simulink library "StatemachineMARCH"  (R2016b)
settings: Solver=VariableStepAuto  StartTime=0.0  StopTime=10.0  RelTol=1e-3
settings Model: Creator=Nathan  LastModifiedBy=march

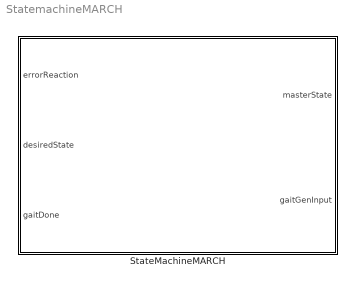
== system StatemachineMARCH ==
  StateMachineMARCH : Stateflow chart  TreatAsAtomicUnit=on

== stateflow chart StatemachineMARCH/StateMachineMARCH ==
  state MASTER_SHUTDOWN
    en: masterState = ExoskeletonState.SHUTTING_DOWN;
  state OPERATION
    state SLOPEUP
      en: masterState = ExoskeletonState.SLOPEUP;
      state startRightSlopeUp
        en: gaitGenInput.targetLeg = Leg.RIGHT;
        %Both leg vectors play at the same time so this only determines
        %what leg starts the stairs step.
        % Leg.Right = Right leg starts stairs step
        % Leg.Left = Left leg starts stair step
        en: gaitGenInput.stepType = StepType.SLOPEUPSTEP;
      state WAIT_SLOPEUP
        en: masterState = ExoskeletonState.SLOPEUP;
        en: gaitGenInput.stepType = StepType.WAITSLOPEUP;
        en: gaitGenInput.targetLeg = Leg.BOTH;
      state INITIALIZE_SLOPEUP
        en: masterState = ExoskeletonState.SLOPEUP;
        en: gaitGenInput.stepType = StepType.INITIALIZESLOPEUP;
        en: gaitGenInput.targetLeg = Leg.BOTH;
      WAIT_SLOPEUP -> startRightSlopeUp [order 1] : [gaitDone]
      INITIALIZE_SLOPEUP -> WAIT_SLOPEUP : [gaitDone]
    state FULLMANUAL
      en: masterState = ExoskeletonState.FULLMANUAL;
    state MANUAL
      en: masterState = ExoskeletonState.MANUAL;
      en: gaitGenInput.targetLeg=Leg.NONE;
      en: gaitGenInput.stepType=StepType.NOSTEP;
    state HOLDSOFA
      en: masterState = ExoskeletonState.HOLDSOFA;
      en: gaitGenInput.stepType = StepType.HOMESOFA;
      en: gaitGenInput.targetLeg = Leg.BOTH;
    state HOLDSIT
      en: masterState = ExoskeletonState.HOLDSIT;
      en: gaitGenInput.stepType = StepType.HOMESIT;
      en: gaitGenInput.targetLeg = Leg.BOTH;
    state STANDUPPROCEDURE
      state INITIALIZE_STANDUP
        en: masterState = ExoskeletonState.STANDINGUP;
        en: gaitGenInput.stepType = StepType.INITIALIZESTANDUP;
        en: gaitGenInput.targetLeg = Leg.BOTH;
      state WAIT_STANDUP
        en: masterState = ExoskeletonState.STANDINGUP;
        en: gaitGenInput.stepType = StepType.WAITSTANDUP;
        en: gaitGenInput.targetLeg = Leg.BOTH;
      state STANDUP
        en: masterState = ExoskeletonState.STANDINGUP;
        en: gaitGenInput.stepType = StepType.STANDUP;
        en: gaitGenInput.targetLeg = Leg.BOTH;
      INITIALIZE_STANDUP -> WAIT_STANDUP : [gaitDone]
      WAIT_STANDUP -> STANDUP [order 2] : [desiredState==ExoskeletonState.HOLDSTAND & gaitDone]
    state SITDOWNPROCEDURE
      state SITDOWN
        en: masterState = ExoskeletonState.SITTINGDOWN;
        en: gaitGenInput.stepType = StepType.SITDOWN;
        en: gaitGenInput.targetLeg = Leg.BOTH;
      state WAIT_SITDOWN
        en: masterState = ExoskeletonState.SITTINGDOWN;
        en: gaitGenInput.stepType = StepType.WAITSITDOWN;
        en: gaitGenInput.targetLeg = Leg.BOTH;
      state INITIALIZE_SITDOWN
        en: masterState = ExoskeletonState.SITTINGDOWN;
        en: gaitGenInput.stepType = StepType.INITIALIZESITDOWN;
        en: gaitGenInput.targetLeg = Leg.BOTH;
      WAIT_SITDOWN -> SITDOWN [order 1] : [desiredState==ExoskeletonState.HOLDSIT & gaitDone]
      INITIALIZE_SITDOWN -> WAIT_SITDOWN : [gaitDone]
    state SOFADOWNPROCEDURE
      state SOFADOWN
        en: masterState = ExoskeletonState.SOFADOWN;
        en: gaitGenInput.stepType = StepType.SOFADOWNSTEP;
        en: gaitGenInput.targetLeg = Leg.BOTH;
      state WAIT_SOFADOWN
        en: masterState = ExoskeletonState.SOFADOWN;
        en: gaitGenInput.stepType = StepType.WAITSOFADOWN;
        en: gaitGenInput.targetLeg = Leg.BOTH;
      state INITIALIZE_SOFADOWN
        en: masterState = ExoskeletonState.SOFADOWN;
        en: gaitGenInput.stepType = StepType.INITIALIZESOFADOWN;
        en: gaitGenInput.targetLeg = Leg.BOTH;
      WAIT_SOFADOWN -> SOFADOWN : [gaitDone]
      INITIALIZE_SOFADOWN -> WAIT_SOFADOWN : [gaitDone]
    state SOFAUPPROCEDURE
      state INITIALIZE_SOFAUP
        en: masterState = ExoskeletonState.SOFAUP;
        en: gaitGenInput.stepType = StepType.INITIALIZESOFAUP;
        en: gaitGenInput.targetLeg = Leg.BOTH;
      state WAIT_SOFAUP
        en: masterState = ExoskeletonState.SOFAUP;
        en: gaitGenInput.stepType = StepType.WAITSOFAUP;
        en: gaitGenInput.targetLeg = Leg.BOTH;
      state SOFAUP
        en: masterState = ExoskeletonState.SOFAUP;
        en: gaitGenInput.stepType = StepType.SOFAUPSTEP;
        en: gaitGenInput.targetLeg = Leg.BOTH;
      INITIALIZE_SOFAUP -> WAIT_SOFAUP : [gaitDone]
      WAIT_SOFAUP -> SOFAUP : [gaitDone]
    state SLOPEDOWN
      en: masterState = ExoskeletonState.SLOPEDOWN;
      state INITIALIZE_SLOPEDOWN
        en: masterState = ExoskeletonState.SLOPEDOWN;
        en: gaitGenInput.stepType = StepType.INITIALIZESLOPEDOWN;
        en: gaitGenInput.targetLeg = Leg.BOTH;
      state WAIT_SLOPEDOWN
        en: masterState = ExoskeletonState.SLOPEDOWN;
        en: gaitGenInput.stepType = StepType.WAITSLOPEDOWN;
        en: gaitGenInput.targetLeg = Leg.BOTH;
      state startRightSLOPEDown
        en: gaitGenInput.targetLeg = Leg.RIGHT;
        %Both leg vectors play at the same time so this only determines
        %what leg starts the stairs step.
        % Leg.Right = Right leg starts stairs step
        % Leg.Left = Left leg starts stair step
        en: gaitGenInput.stepType = StepType.SLOPEDOWNSTEP;
      INITIALIZE_SLOPEDOWN -> WAIT_SLOPEDOWN : [gaitDone]
      WAIT_SLOPEDOWN -> startRightSLOPEDown [order 1] : [gaitDone]
    state HOLDSTAND
      en: masterState = ExoskeletonState.HOLDSTAND;
      en: gaitGenInput.stepType = StepType.HOMESTAND;
      en: gaitGenInput.targetLeg = Leg.BOTH;
    state CONTINUOUSGAIT
      en: masterState = ExoskeletonState.CONTINUOUSGAIT;
      state makeRightHalfStepCont
        en: gaitGenInput.targetLeg = Leg.RIGHT;
        en: gaitGenInput.stepType = StepType.HALFSTEPSTOP;
      state makeLeftHalfStepCont
        en: gaitGenInput.targetLeg = Leg.LEFT;
        en: gaitGenInput.stepType = StepType.HALFSTEPSTOP;
      state finishLeftFullStepCont
        % exoskeleton finishes left step
      state finishRightFullStepCont
        % exoskeleton finishes right step
      state startRightHalfStepCont
        en: gaitGenInput.targetLeg = Leg.RIGHT;
        en: gaitGenInput.stepType = StepType.HALFSTEPSTART;
      state rightFullStepCont
        en: gaitGenInput.targetLeg = Leg.RIGHT;
        en: gaitGenInput.stepType = StepType.FULLSTEP;
      state leftFullStepCont
        en: gaitGenInput.targetLeg = Leg.LEFT;
        en: gaitGenInput.stepType = StepType.FULLSTEP;
      finishLeftFullStepCont -> makeRightHalfStepCont : [gaitDone]
      finishRightFullStepCont -> makeLeftHalfStepCont : [gaitDone]
      startRightHalfStepCont -> finishRightFullStepCont [order 2] : [desiredState ~= ExoskeletonState.CONTINUOUSGAIT]
      startRightHalfStepCont -> leftFullStepCont [order 1] : [gaitDone]
      rightFullStepCont -> finishRightFullStepCont [order 1] : [desiredState ~= ExoskeletonState.CONTINUOUSGAIT]
      leftFullStepCont -> finishLeftFullStepCont [order 1] : [desiredState ~= ExoskeletonState.CONTINUOUSGAIT]
      leftFullStepCont -> rightFullStepCont [order 2] : [gaitDone]
      rightFullStepCont -> leftFullStepCont [order 2] : [gaitDone]
    state STAIRSUP
      en: masterState = ExoskeletonState.STAIRSUP;
      state startRightStairsUp
        en: gaitGenInput.targetLeg = Leg.RIGHT;
        %Both leg vectors play at the same time so this only determines
        %what leg starts the stairs step.
        % Leg.Right = Right leg starts stairs step
        % Leg.Left = Left leg starts stair step
        en: gaitGenInput.stepType = StepType.STAIRSUPSTEP;
      state WAIT_STAIRSUP
        en: masterState = ExoskeletonState.STAIRSUP;
        en: gaitGenInput.stepType = StepType.WAITSTAIRSUP;
        en: gaitGenInput.targetLeg = Leg.BOTH;
      state INITIALIZE_STAIRSUP
        en: masterState = ExoskeletonState.STAIRSUP;
        en: gaitGenInput.stepType = StepType.INITIALIZESTAIRSUP;
        en: gaitGenInput.targetLeg = Leg.BOTH;
      WAIT_STAIRSUP -> startRightStairsUp : [gaitDone]
      INITIALIZE_STAIRSUP -> WAIT_STAIRSUP : [gaitDone]
    state STAIRSDOWN
      en: masterState = ExoskeletonState.STAIRSDOWN;
      state INITIALIZE_STAIRSDOWN
        en: masterState = ExoskeletonState.STAIRSDOWN;
        en: gaitGenInput.stepType = StepType.INITIALIZESTAIRSDOWN;
        en: gaitGenInput.targetLeg = Leg.BOTH;
      state WAIT_STAIRSDOWN
        en: masterState = ExoskeletonState.STAIRSDOWN;
        en: gaitGenInput.stepType = StepType.WAITSTAIRSDOWN;
        en: gaitGenInput.targetLeg = Leg.BOTH;
      state startRightStairsDown
        en: gaitGenInput.targetLeg = Leg.RIGHT;
        %Both leg vectors play at the same time so this only determines
        %what leg starts the stairs step.
        % Leg.Right = Right leg starts stairs step
        % Leg.Left = Left leg starts stair step
        en: gaitGenInput.stepType = StepType.STAIRSDOWNSTEP;
      INITIALIZE_STAIRSDOWN -> WAIT_STAIRSDOWN : [gaitDone]
      WAIT_STAIRSDOWN -> startRightStairsDown : [gaitDone]
    state ROUGHTERRAIN
      en: masterState = ExoskeletonState.ROUGHTERRAIN;
      state roughTerrainStep
        en: gaitGenInput.targetLeg = Leg.RIGHT;
        en: gaitGenInput.stepType = StepType.ROUGHTERRAINSTEP;
    (default) -> MANUAL
    HOLDSOFA -> MANUAL [order 2] : [desiredState==ExoskeletonState.MANUAL && gaitDone]
    FULLMANUAL -> HOLDSOFA [order 4] : [desiredState==ExoskeletonState.HOLDSOFA]
    MANUAL -> FULLMANUAL [order 1] : [gaitDone]
    FULLMANUAL -> HOLDSIT [order 2] : [desiredState==ExoskeletonState.HOLDSIT]
    FULLMANUAL -> HOLDSTAND [order 1] : [desiredState==ExoskeletonState.HOLDSTAND]
    HOLDSIT -> MANUAL [order 1] : [desiredState==ExoskeletonState.MANUAL && gaitDone]
    startRightSlopeUp -> HOLDSTAND : [[desiredState ~= Exoskeleton.SLOPEUP && gaitDone]]
    SOFADOWN -> HOLDSOFA : [gaitDone]
    HOLDSOFA -> INITIALIZE_SOFAUP [order 1] : [desiredState==ExoskeletonState.HOLDSTAND & gaitDone]
    WAIT_SLOPEUP -> HOLDSTAND [order 2] : [desiredState ~= Exoskeleton.SLOPEUP]
    WAIT_STANDUP -> HOLDSIT [order 1] : [desiredState~=ExoskeletonState.HOLDSTAND]
    SITDOWN -> HOLDSIT : [gaitDone]
    HOLDSIT -> INITIALIZE_STANDUP [order 3] : [desiredState==ExoskeletonState.HOLDSTAND & gaitDone]
    HOLDSTAND -> INITIALIZE_SLOPEUP [order 6] : [desiredState==ExoskeletonState.SLOPEUP && gaitDone]
    WAIT_SITDOWN -> HOLDSTAND [order 2] : [desiredState ~= ExoskeletonState.HOLDSIT]
    HOLDSTAND -> INITIALIZE_SLOPEDOWN [order 5] : [desiredState==ExoskeletonState.SLOPEDOWN && gaitDone]
    STANDUP -> HOLDSTAND : [gaitDone]
    HOLDSTAND -> INITIALIZE_SITDOWN [order 2] : [desiredState==ExoskeletonState.HOLDSIT && gaitDone]
    HOLDSTAND -> INITIALIZE_SOFADOWN [order 7] : [desiredState==ExoskeletonState.HOLDSOFA && gaitDone]
    SOFAUP -> HOLDSTAND : [gaitDone]
    WAIT_SLOPEDOWN -> HOLDSTAND [order 2] : [desiredState ~= Exoskeleton.SLOPEDOWN]
    startRightSLOPEDown -> HOLDSTAND : [desiredState ~= Exoskeleton.SLOPEDOWN && gaitDone]
    makeRightHalfStepCont -> HOLDSTAND : [gaitDone]
    HOLDSTAND -> startRightHalfStepCont [order 3] : [desiredState==ExoskeletonState.CONTINUOUSGAIT && gaitDone]
    makeLeftHalfStepCont -> HOLDSTAND : [gaitDone]
    startRightStairsUp -> HOLDSTAND : [gaitDone]
    HOLDSTAND -> INITIALIZE_STAIRSDOWN [order 1] : [desiredState==ExoskeletonState.STAIRSDOWN && gaitDone]
    startRightStairsDown -> HOLDSTAND : [gaitDone]
    roughTerrainStep -> HOLDSTAND : [gaitDone]
    HOLDSTAND -> roughTerrainStep [order 8] : [desiredState==ExoskeletonState.ROUGHTERRAIN && gaitDone]
    HOLDSTAND -> INITIALIZE_STAIRSUP [order 4] : [desiredState==ExoskeletonState.STAIRSUP && gaitDone]
  state SEVERE_ERROR
    en: masterState = ExoskeletonState.SEVERE_ERROR;
  SEVERE_ERROR -> MASTER_SHUTDOWN [order 2] : [desiredState==ExoskeletonState.SHUTTING_DOWN]
  (default) -> OPERATION
  FULLMANUAL -> MASTER_SHUTDOWN [order 3] : [desiredState==ExoskeletonState.SHUTTING_DOWN]
  MANUAL -> MASTER_SHUTDOWN [order 2] : [desiredState==ExoskeletonState.SHUTTING_DOWN]
  HOLDSIT -> MASTER_SHUTDOWN [order 2] : [desiredState==ExoskeletonState.SHUTTING_DOWN]
  OPERATION -> SEVERE_ERROR : [errorReaction == ErrorReaction.QUITIMMEDIATELY]
  SEVERE_ERROR -> OPERATION [order 1] : [errorReaction == ErrorReaction.NOREACTION]
  data: masterState output Enum: ExoskeletonState; errorReaction input Enum: ErrorReaction; desiredState input; gaitDone input; gaitGenInput output Bus: GaitGeneratorInput
